simulink model "Project_Model_3"  (Simulink 7.9)
settings: Solver=ode3  StartTime=0.0  StopTime=80  FixedStep=0.001  RelTol=1e-3
values from neighbouring files (symbols this model uses):
  d_cm = 10    [Project_Model_Params.m]
  den = [1 5.18 14.12]    [Project_Model_Params.m]    (also in Ziegler_Nichols_0.m = [0.05 1.7185 16.71 49.88 61.35 0]; step_test_params.m = [1 14.37 46.82 61.35])
  duty_max = 100    [Project_Model_Params.m]
  duty_min = 0    [Project_Model_Params.m]
  FF = 30    [Project_Model_Params.m]
  init_d = 12    [Project_Model_Params.m]
  int_max = 150    [Project_Model_Params.m]    (also in step_test_params.m = 1000)
  int_min = -150    [Project_Model_Params.m]    (also in step_test_params.m = -1000)
  Kd = Kp*0.125*P_cr    (= 0.532770091731)    [Project_Model_Params.m]    (also in Ziegler_Nichols_0.m = 0.762550216826; step_test_params.m = 0.955086194687)
  Ki = Kp*2/P_cr    (= 2.12892018077)    [Project_Model_Params.m]    (also in Ziegler_Nichols_0.m = 4.58089306504; step_test_params.m = 3.46055049103)
  Kp = 0.6*K_cr    (= 2.13)    [Project_Model_Params.m]    (also in Ziegler_Nichols_0.m = 3.738; step_test_params.m = 3.636)
  lead_v = 30    [Project_Model_Params.m]
  num = [15.12]    [Project_Model_Params.m]    (also in Ziegler_Nichols_0.m = [-0.803 13.874 43.72]; step_test_params.m = [16.06 43.72])
  offset = -20    [Project_Model_Params.m]
  Ts = 0.1    [Project_Model_Params.m]    (also in step_test_params.m)
settings Model: Creator=ipd501  LastModifiedBy=quchao
settings GRTTargetCC: CombineOutputUpdateFcns=off  GRTInterface=on

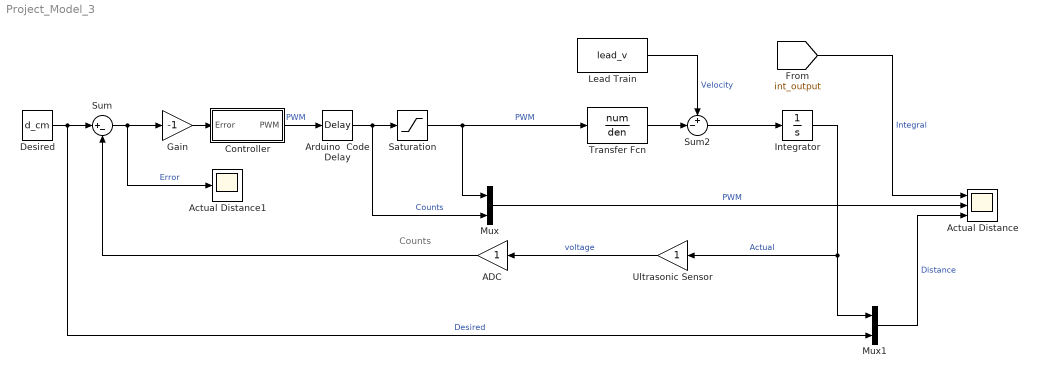
== system Project_Model_3 ==
  note: Counts
  ADC : Gain
  Actual Distance : Scope  NumInputPorts=3
      settings: TimeRange=80  YMin=-5~-5~-5  YMax=5~5~5
  Actual Distance1 : Scope
  Arduino  Code Delay : TransportDelay  DelayTime=Ts
  Controller : Subsystem
  Desired : Constant  Value=d_cm
  Gain : Gain  Gain=-1
  Integrator : Integrator  InitialCondition=init_d
  Lead Train : Constant  Value=lead_v
  Mux : Mux  Inputs=2
  Mux1 : Mux  Inputs=2
  Saturation : Saturate  UpperLimit=duty_max  LowerLimit=duty_min
  Sum : Sum  Inputs=|+-
  Sum2 : Sum  Inputs=+-|
  Transfer Fcn : TransferFcn  Numerator=num  Denominator=den
  Ultrasonic Sensor : Gain
  wires:
  ADC/1 -> Sum/2
  Sum2/1 -> Integrator/1
  Integrator/1 -> Ultrasonic Sensor/1, Mux1/1  "Actual"
  Ultrasonic Sensor/1 -> ADC/1  "voltage"
  Saturation/1 -> Transfer Fcn/1, Mux/1  "PWM"
  Controller/1(PWM) -> Arduino  Code Delay/1  "PWM"
  Transfer Fcn/1 -> Sum2/2
  Lead Train/1 -> Sum2/1  "Velocity"
  Desired/1 -> Sum/1, Mux1/2  "Desired"
  Sum/1 -> Gain/1, Actual Distance1/1  "Error"
  [int_output] -> Actual Distance/1  "Integral"
  Mux1/1 -> Actual Distance/3  "Distance"
  Mux/1 -> Actual Distance/2  "PWM"
  Gain/1 -> Controller/1(Error)
  Arduino  Code Delay/1 -> Saturation/1, Mux/2  "Counts"

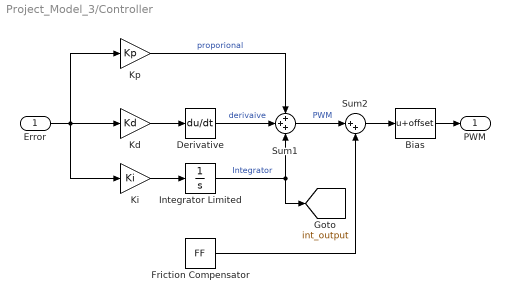
== system Project_Model_3/Controller ==
  Error : Inport
  Bias : Bias  Bias=offset
  Derivative : Derivative
  Friction Compensator : Constant  Value=FF
  Integrator Limited : Integrator  LimitOutput=on  UpperSaturationLimit=int_max  LowerSaturationLimit=int_min
  Kd : Gain  Gain=Kd
  Ki : Gain  Gain=Ki
  Kp : Gain  Gain=Kp
  Sum1 : Sum  Inputs=+++
  Sum2 : Sum  Inputs=|++
  PWM : Outport
  tag scope: int_output=global
  wires:
  Kd/1 -> Derivative/1
  Ki/1 -> Integrator Limited/1
  Kp/1 -> Sum1/1  "proporional"
  Derivative/1 -> Sum1/2  "derivaive"
  Integrator Limited/1 -> Sum1/3, [int_output]  "Integrator"
  Error/1 -> Ki/1, Kp/1, Kd/1
  Bias/1 -> PWM/1
  Sum1/1 -> Sum2/1  "PWM"
  Sum2/1 -> Bias/1
  Friction Compensator/1 -> Sum2/2
